simulink model "sgMdl_ARINC825_Loopback"  (R2024b)
settings: Solver=FixedStepAuto  StartTime=0.0  StopTime=inf  RelTol=1e-3
undefined symbols (not defined in the file): IO602
libraries: speedgoatlib_ARINC825 x5, slrealtimeutilitieslib x4, canfdmsglib x2
Description:
  | ARINC 825 - Loopback
settings Model: ModifiedByFormat=Speedgoat  Creator=Speedgoat  LastModifiedBy=Speedgoat
settings SolverCC: ConcurrentTasks=on  AlgebraicLoopSolver=TrustRegion  PositivePriorityOrder=on  AutoInsertRateTranBlk=on
settings OptimizationCC: BlockReduction=off  OptimizeBlockIOStorage=off
settings DebuggingCC: TasksWithSamePriorityMsg=none  UnconnectedInputMsg=warning  UnconnectedOutputMsg=warning  UnconnectedLineMsg=warning
settings HardwareCC: ProdBitPerLong=64  ProdLongLongMode=on  ProdHWDeviceType=Intel->x86-64 (Linux 64)
settings ModelReferenceCC: EnableRefExpFcnMdlSchedulingChecks=on
settings RTWCC: Description=Speedgoat Real-Time Target Machine  SystemTargetFile=speedgoat.tlc  TemplateMakefile=slrealtime_default_tmf  Toolchain=Simulink Real-Time Toolchain  BuildConfiguration=Faster Runs  TargetLang=C++  GPUComputeCapability=3.5  DLArmComputeVersion=19.05
settings SimulinkRealTimeTargetCC: SubcomponentCodeInterfacePackaging=Reusable function  InstructionSetFMA=off  LogToMDFFile=off  SLRTFileLogMaxRuns=10  UseGCCFastMath=on
settings ConfigComp: CovBoundaryAbsTol=1.0e-5

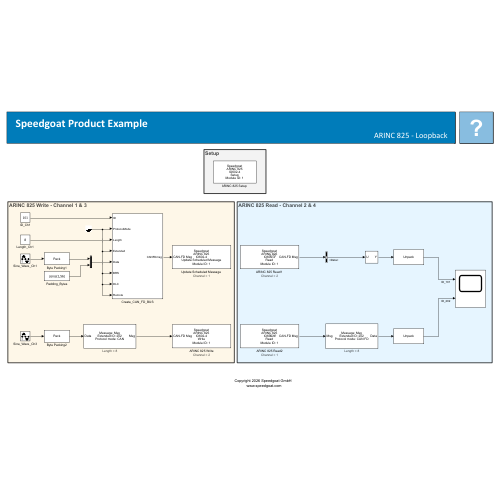
[thumbnail: Simulink's stored preview of the top-level diagram]
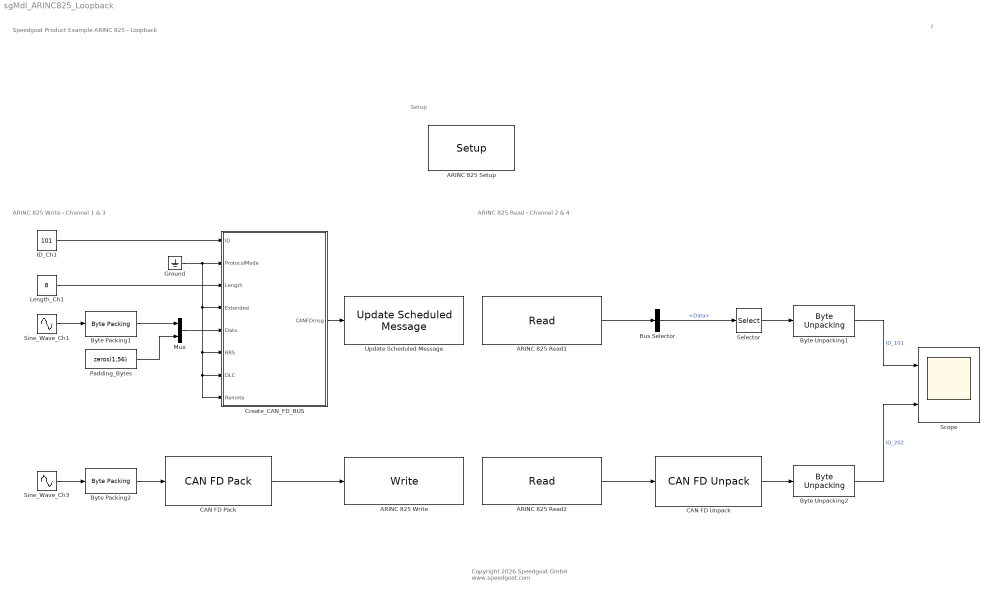
== system sgMdl_ARINC825_Loopback ==
  note: ARINC 825 Write - Channel 1 & 3
  note: Setup
  note: ARINC 825 Read - Channel 2 & 4
  note: Speedgoat Product Example
      | ARINC 825 - Loopback
  note: ?
  note: Copyright 2026 Speedgoat GmbH
      |  www.speedgoat.com
  "ARINC 825 Read1 " : speedgoatlib_ARINC825/Read   parModuleType=IO602-2  parModuleId=1  parChannel=2  parMessageId=[101]  parSampleTime=0.01  parEnInput=off  parStatusOutput=off  parPciSlot=-1
      settings: AttributesFormatString=Channel = %<parChannel>  SourceProductName=Simulink Real-Time: Speedgoat I/O Blockset
  ARINC 825 Read2 : speedgoatlib_ARINC825/Read   parModuleType=IO602-2  parModuleId=1  parChannel=1  parMessageId=[202]  parSampleTime=0.01  parEnInput=off  parStatusOutput=off  parPciSlot=-1
      settings: AttributesFormatString=Channel = %<parChannel>  SourceProductName=Simulink Real-Time: Speedgoat I/O Blockset
  "ARINC 825 Setup " : speedgoatlib_ARINC825/Setup   parModuleType=IO602-2  parModuleId=1  parPciSlot=-1  parEnableCh1=CAN (HS)  parEnableCh2=CAN (HS)  parEnableCh3=Disabled  parEnableCh4=Disabled  parAllowCAN=off  parBaudCh1=1000  parCustomBaudCh1=10  parBaudFDCh1=5000  parCustomBaudFDCh1=[2, 2, 5, 2]  parBaudCh2=1000  parCustomBaudCh2=10  parBaudFDCh2=5000  parCustomBaudFDCh2=[2, 2, 5, 2]  parBaudCh3=1000  parCustomBaudCh3=10  parBaudFDCh3=5000  parCustomBaudFDCh3=[2, 2, 5, 2]  parBaudCh4=1000  parCustomBaudCh4=10  parBaudFDCh4=5000  parCustomBaudFDCh4=[2, 2, 5, 2]  parModeSchedMsg=Manual  parTicksCh1=800000  parIntervalCh1=0.01  parSchedMsgCh1=[101 8 41 92 143 194 245 40 172 63 0 0 0 0 0 0 0 0 0 0 0 0 0 0 0 0 0 0 0 0 0 0 0 0 0 0 0 0 0 0 0 0 0 0 0 0 0 0 0 0 0 0 0 0 0 0 0 0 0 0 0 0 0 0 0 0 1 1 0.05 0]  parSchedMsgNameCh1={'Message1'}  parTicksCh2=800000  parIntervalCh2=0.01  parSchedMsgCh2=0  parSchedMsgNameCh2=0  parTicksCh3=80000  parIntervalCh3=0.001  parSchedMsgCh3=0  parSchedMsgNameCh3=0  parTicksCh4=80000  parIntervalCh4=0.001  parSchedMsgCh4=0  parSchedMsgNameCh4=0  parSchedMsgConfigFile=''
      settings: SourceProductName=Simulink Real-Time: Speedgoat I/O Blockset
  ARINC 825 Write : speedgoatlib_ARINC825/Write   parModuleType=IO602-2  parModuleId=1  parChannel=2  parInWidth=1  parSampleTime=0.1  parEnInput=off  parPciSlot=-1
      settings: AttributesFormatString=Channel = %<parChannel>  SourceProductName=Simulink Real-Time: Speedgoat I/O Blockset
  Bus Selector : BusSelector  OutputSignals=Data
  Byte Packing1 : slrealtimeutilitieslib/Byte Packing  MaskPackedDataType=uint8  MaskUnpackedDataTypes={'double'}  MaskAlignment=1
  Byte Packing2 : slrealtimeutilitieslib/Byte Packing  MaskPackedDataType=uint8  MaskUnpackedDataTypes={'double'}  MaskAlignment=1
  Byte Unpacking1 : slrealtimeutilitieslib/Byte Unpacking  MaskUnpackedDataTypes={'double'}  MaskUnpackedDataSizes={[1]}  MaskAlignment=1
  Byte Unpacking2 : slrealtimeutilitieslib/Byte Unpacking  MaskUnpackedDataTypes={'double'}  MaskUnpackedDataSizes={[1]}  MaskAlignment=1
  CAN FD Pack : canfdmsglib/CAN FD Pack  MsgList=(none)  MsgName=Msg  ProtocolMode=CAN  MsgIDType=Extended (29-bit identifier)  MsgIdentifier=202  CANIDInput=off  MsgLength=8  Remote=off  BRSSwitch=off  ApplyMinMax=off  SignalInfo={}
      settings: AttributesFormatString=Length = %<MsgLength>  DataFormat=raw data
  CAN FD Unpack : canfdmsglib/CAN FD Unpack  MsgList=(none)  MsgName=Msg  ProtocolMode=CAN FD  MsgIDType=Extended (29-bit identifier)  MsgIdentifier=202  MsgLength=8  SignalInfo={}  IDPort=off  TimestampPort=off  ErrorPort=off  RemotePort=off  LengthPort=off  StatusPort=off  BRSPort=off  ESIPort=off  DLCPort=off  ApplyMinMax=off
      settings: AttributesFormatString=Length = %<MsgLength>  DataFormat=raw data
  Create_CAN_FD_BUS : Subsystem
  Ground : Ground
  ID_Ch1 : Constant  Value=101  OutDataTypeStr=Inherit: Inherit via back propagation  SampleTime=0.05
  Length_Ch1 : Constant  Value=8  OutDataTypeStr=Inherit: Inherit via back propagation  SampleTime=0.05
  Mux : Mux  Inputs=2
  Padding_Bytes : Constant  Value=zeros(1,56)  OutDataTypeStr=Inherit: Inherit via back propagation  SampleTime=-1
  Scope : Scope  NumInputPorts=2
  Selector : Selector  InputPortWidth=64  IndexOptions=Index vector (dialog)  Indices=[1:8]  OutputSizes=1
  Sine_Wave_Ch1 : Sin  SineType=Sample based  Amplitude=10  Bias=10  Frequency=1*2*pi  Samples=100  SampleTime=0.05
  Sine_Wave_Ch3 : Sin  SineType=Sample based  Amplitude=10  Frequency=1*2*pi  Samples=50  SampleTime=0.1
  "Update Scheduled Message " : speedgoatlib_ARINC825/Update Scheduled Message   parModuleType=IO602-2  parModuleId=1  parChannel=1  parMessageId=101  parSampleTime=0.05  parEnInput=off  parPciSlot=-1
      settings: AttributesFormatString=Channel = %<parChannel>  SourceProductName=Simulink Real-Time: Speedgoat I/O Blockset
  wires:
  "ARINC 825 Read1 "/1 -> Bus Selector/1
  Create_CAN_FD_BUS/1(CANFDmsg) -> "Update Scheduled Message "/1
  Bus Selector/1 -> Selector/1  "<Data>"
  Sine_Wave_Ch1/1 -> Byte Packing1/1
  Sine_Wave_Ch3/1 -> Byte Packing2/1
  Byte Unpacking1/1 -> Scope/1  "ID_101"
  CAN FD Unpack/1 -> Byte Unpacking2/1
  CAN FD Pack/1 -> ARINC 825 Write/1
  Byte Packing2/1 -> CAN FD Pack/1
  ARINC 825 Read2/1 -> CAN FD Unpack/1
  ID_Ch1/1 -> Create_CAN_FD_BUS/1(ID)
  Length_Ch1/1 -> Create_CAN_FD_BUS/3(Length)
  Mux/1 -> Create_CAN_FD_BUS/5(Data)
  Byte Packing1/1 -> Mux/1
  Padding_Bytes/1 -> Mux/2
  Selector/1 -> Byte Unpacking1/1
  Byte Unpacking2/1 -> Scope/2  "ID_202"
  Ground/1 -> Create_CAN_FD_BUS/8(Remote), Create_CAN_FD_BUS/7(DLC), Create_CAN_FD_BUS/6(BRS), Create_CAN_FD_BUS/4(Extended), Create_CAN_FD_BUS/2(ProtocolMode)

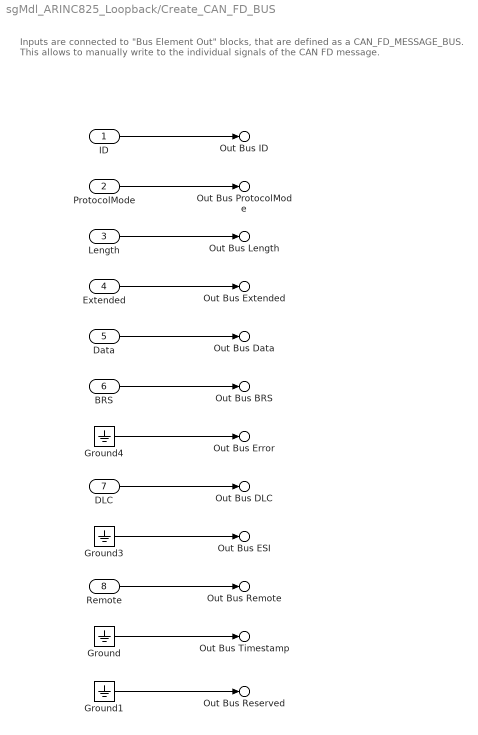
== system sgMdl_ARINC825_Loopback/Create_CAN_FD_BUS ==
  note: Inputs are connected to "Bus Element Out" blocks, that are defined as a CAN_FD_MESSAGE_BUS.
      | This allows to manually write to the individual signals of the CAN FD message.
  ID : Inport
  ProtocolMode : Inport  Port=2
  Length : Inport  Port=3
  Extended : Inport  Port=4
  Data : Inport  Port=5
  BRS : Inport  Port=6
  DLC : Inport  Port=7
  Remote : Inport  Port=8
  Ground{,1,3..4} (4 alike) : Ground
  Out Bus ProtocolMode : Outport  PortName=CANFDmsg  Element=ProtocolMode
  Out Bus Extended : Outport  PortName=CANFDmsg  Element=Extended
  Out Bus Length : Outport  PortName=CANFDmsg  Element=Length
  Out Bus Remote : Outport  PortName=CANFDmsg  Element=Remote
  Out Bus Error : Outport  PortName=CANFDmsg  Element=Error
  Out Bus BRS : Outport  PortName=CANFDmsg  Element=BRS
  Out Bus ESI : Outport  PortName=CANFDmsg  Element=ESI
  Out Bus DLC : Outport  PortName=CANFDmsg  Element=DLC
  Out Bus ID : Outport  PortName=CANFDmsg  Element=ID
  Out Bus Reserved : Outport  PortName=CANFDmsg  Element=Reserved
  Out Bus Timestamp : Outport  PortName=CANFDmsg  Element=Timestamp
  Out Bus Data : Outport  PortName=CANFDmsg  Element=Data
  wires:
  ID/1 -> Out Bus ID/1
  ProtocolMode/1 -> Out Bus ProtocolMode/1
  Length/1 -> Out Bus Length/1
  Extended/1 -> Out Bus Extended/1
  Data/1 -> Out Bus Data/1
  BRS/1 -> Out Bus BRS/1
  Ground4/1 -> Out Bus Error/1
  DLC/1 -> Out Bus DLC/1
  Ground3/1 -> Out Bus ESI/1
  Remote/1 -> Out Bus Remote/1
  Ground/1 -> Out Bus Timestamp/1
  Ground1/1 -> Out Bus Reserved/1
